simulink model "PID_Simulation_System_A"  (R2018b)
settings: Solver=VariableStepAuto  StartTime=0.0  StopTime=10  RelTol=1e-3
undefined symbols (not defined in the file): B, b, g, h, Jeq, k_noise, Kb, kd, ki, Km, kp, l, La, M, m, N, r, Ra
libraries: simulink x5, simulink_extras x1
settings Model: Creator=fred  LastModifiedBy=fredericovaz
settings SolverCC: AlgebraicLoopSolver=LineSearch
settings HardwareCC: ProdBitPerLong=64  ProdHWDeviceType=Intel->x86-64 (Linux 64)

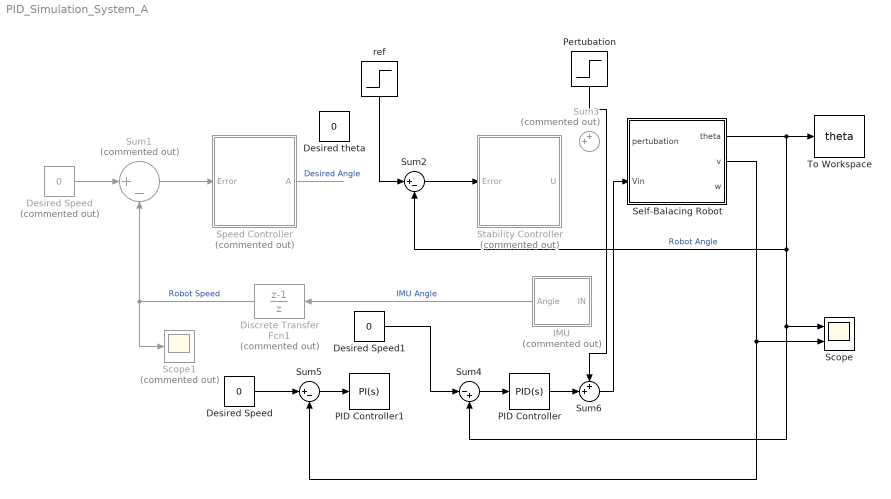
== system PID_Simulation_System_A ==
  Desired Speed : Constant  Value=0
  "Desired Speed " : Constant  Commented=on  Value=0
  Desired Speed1 : Constant  Value=0
  "Desired theta " : Constant  Value=0
  Discrete Transfer Fcn1 : DiscreteTransferFcn  Commented=on  Numerator=[1 -1]  Denominator=[1 0]  SampleTime=h
  IMU : Subsystem  Commented=on
  PID Controller : simulink/Continuous/PID Controller  Controller=PID  Form=Parallel  TimeDomain=Continuous-time  SampleTime=-1  IntegratorMethod=Forward Euler  FilterMethod=Forward Euler  ControllerParametersSource=internal  P=3218.54164072839  I=409.836899495035  D=13019.6852840674  UseFilter=on  N=3228.39836467521  TunerSelectOption=Transfer Function Based (PID Tuner App)  InitialConditionSource=internal  InitialConditionForIntegrator=0  InitialConditionForFilter=0  DifferentiatorICPrevScaledInput=0  ExternalReset=none  TrackingMode=off  Kt=1  LimitOutput=off  UpperSaturationLimit=inf  LowerSaturationLimit=-inf  LinearizeAsGain=on  AntiWindupMode=none  Kb=1  POutMin=[]  POutMax=[]  IOutMin=[]  IOutMax=[]  DOutMin=[]  DOutMax=[]  NOutMin=[]  NOutMax=[]  SumOutMin=[]  SumOutMax=[]  SaturationOutMin=[]  SaturationOutMax=[]  PParamMin=[]  PParamMax=[]  IParamMin=[]  IParamMax=[]  DParamMin=[]  DParamMax=[]  NParamMin=[]  NParamMax=[]  KbParamMin=[]  KbParamMax=[]  KtParamMin=[]  KtParamMax=[]  KbOutMin=[]  KbOutMax=[]  KtOutMin=[]  KtOutMax=[]  IntegratorOutMin=[]  IntegratorOutMax=[]  FilterOutMin=[]  FilterOutMax=[]  SumI1OutMin=[]  SumI1OutMax=[]  SumI2OutMin=[]  SumI2OutMax=[]  SumI3OutMin=[]  SumI3OutMax=[]  SumI4OutMin=[]  SumI4OutMax=[]  SumDOutMin=[]  SumDOutMax=[]  DifferentiatorOutMin=[]  DifferentiatorOutMax=[]  FilterDiffOutCoefMin=[]  FilterDiffOutCoefMax=[]  ReciprocalOutMin=[]  ReciprocalOutMax=[]  SumDenOutMin=[]  SumDenOutMax=[]  SumNumOutMin=[]  SumNumOutMax=[]  DivideOutMin=[]  DivideOutMax=[]  IntegratorContinuousStateAttributes=''  IntegratorStateMustResolveToSignalObject=off  IntegratorRTWStateStorageClass=Auto  FilterContinuousStateAttributes=''  FilterStateMustResolveToSignalObject=off  FilterRTWStateStorageClass=Auto  ParallelPVariant=InternalParameters  IdealPVariant=Disabled  IVariant=InternalParameters  DVariant=InternalParameters  IntegratorVariant=Continuous  SatVariant=Disabled  AWVariant=Passthrough  PCopyVariant=Disabled  TRVariant=Disabled  FdbkBlocksVariant=Forward  IdealPFdbkVariant=Disabled  SatFdbkVariant=Disabled  DerivativeFilterVariant=ContFilter  NVariant=InternalParameters  NCopyVariant=Disabled  FilterICVariant=InternalICsFilter  IntegratorICVariant=InternalICs  ExternalResetVariant=Disabled  TRSumVariant=Passthrough  SumFdbkVariant=Disabled  SumVariant=Sum_PID
  PID Controller1 : simulink/Continuous/PID Controller  Controller=PI  Form=Parallel  TimeDomain=Continuous-time  SampleTime=-1  IntegratorMethod=Forward Euler  FilterMethod=Forward Euler  ControllerParametersSource=internal  P=0.000483355764133952  I=1.52555105477767e-06  D=829.68075928854  UseFilter=on  N=20  TunerSelectOption=Transfer Function Based (PID Tuner App)  InitialConditionSource=internal  InitialConditionForIntegrator=0  InitialConditionForFilter=0  DifferentiatorICPrevScaledInput=0  ExternalReset=none  TrackingMode=off  Kt=1  LimitOutput=off  UpperSaturationLimit=inf  LowerSaturationLimit=-inf  LinearizeAsGain=on  AntiWindupMode=none  Kb=1  POutMin=[]  POutMax=[]  IOutMin=[]  IOutMax=[]  DOutMin=[]  DOutMax=[]  NOutMin=[]  NOutMax=[]  SumOutMin=[]  SumOutMax=[]  SaturationOutMin=[]  SaturationOutMax=[]  PParamMin=[]  PParamMax=[]  IParamMin=[]  IParamMax=[]  DParamMin=[]  DParamMax=[]  NParamMin=[]  NParamMax=[]  KbParamMin=[]  KbParamMax=[]  KtParamMin=[]  KtParamMax=[]  KbOutMin=[]  KbOutMax=[]  KtOutMin=[]  KtOutMax=[]  IntegratorOutMin=[]  IntegratorOutMax=[]  FilterOutMin=[]  FilterOutMax=[]  SumI1OutMin=[]  SumI1OutMax=[]  SumI2OutMin=[]  SumI2OutMax=[]  SumI3OutMin=[]  SumI3OutMax=[]  SumI4OutMin=[]  SumI4OutMax=[]  SumDOutMin=[]  SumDOutMax=[]  DifferentiatorOutMin=[]  DifferentiatorOutMax=[]  FilterDiffOutCoefMin=[]  FilterDiffOutCoefMax=[]  ReciprocalOutMin=[]  ReciprocalOutMax=[]  SumDenOutMin=[]  SumDenOutMax=[]  SumNumOutMin=[]  SumNumOutMax=[]  DivideOutMin=[]  DivideOutMax=[]  IntegratorContinuousStateAttributes=''  IntegratorStateMustResolveToSignalObject=off  IntegratorRTWStateStorageClass=Auto  FilterContinuousStateAttributes=''  FilterStateMustResolveToSignalObject=off  FilterRTWStateStorageClass=Auto  ParallelPVariant=InternalParameters  IdealPVariant=Disabled  IVariant=InternalParameters  DVariant=Disabled  IntegratorVariant=Continuous  SatVariant=Disabled  AWVariant=Passthrough  PCopyVariant=Disabled  TRVariant=Disabled  FdbkBlocksVariant=Forward  IdealPFdbkVariant=Disabled  SatFdbkVariant=Disabled  DerivativeFilterVariant=Disabled  NVariant=Disabled  NCopyVariant=Disabled_SignalSpec  FilterICVariant=Disabled  IntegratorICVariant=InternalICs  ExternalResetVariant=Disabled  TRSumVariant=Passthrough  SumFdbkVariant=Disabled  SumVariant=Sum_PI
  Pertubation : Step  Time=2  After=15
  Scope : Scope  NumInputPorts=2
  Scope1 : Scope  Commented=on
  Self-Balacing Robot : Subsystem
  Speed Controller : Subsystem  Commented=on
  Stability Controller : Subsystem  Commented=on
  Sum1 : Sum  Commented=on  Inputs=|+-
  Sum2 : Sum  Inputs=|+-
  Sum3 : Sum  Commented=on  Inputs=++|
  Sum4 : Sum  Inputs=|-+
  Sum5 : Sum  Inputs=|+-
  Sum6 : Sum  Inputs=++|
  To Workspace : ToWorkspace  VariableName=theta  SaveFormat=Timeseries  SampleTime=-1
      settings: Save2DSignal=2-D array (concatenate along first dimension)
  ref : Step  Time=2  After=0.25  SampleTime=h
  wires:
  IMU/1(Angle) -> Discrete Transfer Fcn1/1  "IMU Angle"
  Self-Balacing Robot/1(theta) -> To Workspace/1, Sum2/2, Scope/1, Sum4/2  "Robot Angle"
  Speed Controller/1(A) -> ?  "Desired Angle"
  Sum1/1 -> Speed Controller/1(Error)
  "Desired Speed "/1 -> Sum1/1
  Discrete Transfer Fcn1/1 -> Scope1/1, Sum1/2  "Robot Speed"
  Sum2/1 -> Stability Controller/1(Error)
  ref/1 -> Sum2/1
  Sum4/1 -> PID Controller/1
  Sum5/1 -> PID Controller1/1
  Self-Balacing Robot/2(v) -> Scope/2, Sum5/2
  PID Controller/1 -> Sum6/2
  Sum6/1 -> Self-Balacing Robot/2(Vin)
  Pertubation/1 -> Sum6/1
  Desired Speed/1 -> Sum5/1
  Desired Speed1/1 -> Sum4/1

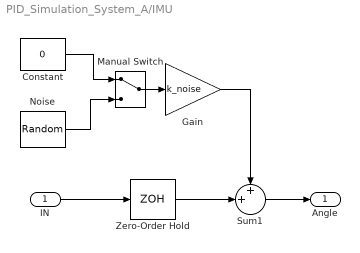
== system PID_Simulation_System_A/IMU ==
  IN : Inport
  Constant : Constant  Value=0
  Gain : Gain  Gain=k_noise
  Manual Switch : ManualSwitch
  Noise : UniformRandomNumber  Minimum=-0.1  Maximum=0.1  SampleTime=h
  Sum1 : Sum  Inputs=++|
  Zero-Order Hold : ZeroOrderHold  SampleTime=h
  Angle : Outport
  wires:
  IN/1 -> Zero-Order Hold/1
  Constant/1 -> Manual Switch/1
  Noise/1 -> Manual Switch/2
  Manual Switch/1 -> Gain/1
  Gain/1 -> Sum1/1
  Zero-Order Hold/1 -> Sum1/2
  Sum1/1 -> Angle/1

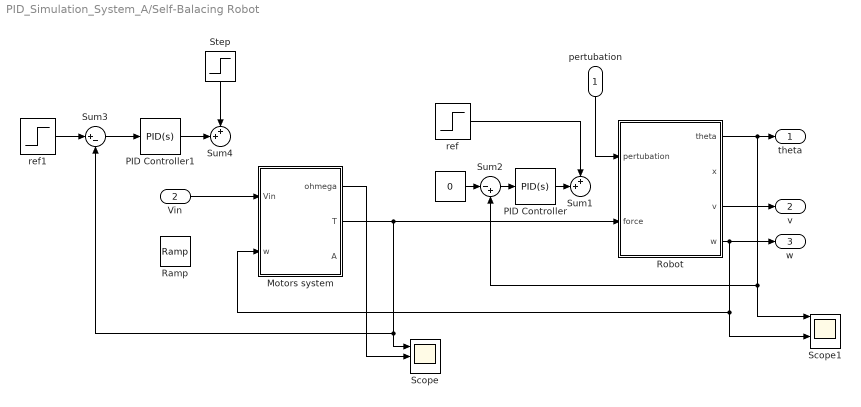
== system PID_Simulation_System_A/Self-Balacing Robot ==
  pertubation : Inport
  Vin : Inport  Port=2
  " " : Constant  Value=0
  Motors system : Subsystem
  PID Controller : simulink/Continuous/PID Controller  Controller=PID  Form=Parallel  TimeDomain=Continuous-time  SampleTime=-1  IntegratorMethod=Forward Euler  FilterMethod=Forward Euler  ControllerParametersSource=internal  P=6572.38369505498  I=1124.56192224529  D=829.68075928854  UseFilter=on  N=20  TunerSelectOption=Transfer Function Based (PID Tuner App)  InitialConditionSource=internal  InitialConditionForIntegrator=0  InitialConditionForFilter=0  DifferentiatorICPrevScaledInput=0  ExternalReset=none  TrackingMode=off  Kt=1  LimitOutput=off  UpperSaturationLimit=inf  LowerSaturationLimit=-inf  LinearizeAsGain=on  AntiWindupMode=none  Kb=1  POutMin=[]  POutMax=[]  IOutMin=[]  IOutMax=[]  DOutMin=[]  DOutMax=[]  NOutMin=[]  NOutMax=[]  SumOutMin=[]  SumOutMax=[]  SaturationOutMin=[]  SaturationOutMax=[]  PParamMin=[]  PParamMax=[]  IParamMin=[]  IParamMax=[]  DParamMin=[]  DParamMax=[]  NParamMin=[]  NParamMax=[]  KbParamMin=[]  KbParamMax=[]  KtParamMin=[]  KtParamMax=[]  KbOutMin=[]  KbOutMax=[]  KtOutMin=[]  KtOutMax=[]  IntegratorOutMin=[]  IntegratorOutMax=[]  FilterOutMin=[]  FilterOutMax=[]  SumI1OutMin=[]  SumI1OutMax=[]  SumI2OutMin=[]  SumI2OutMax=[]  SumI3OutMin=[]  SumI3OutMax=[]  SumI4OutMin=[]  SumI4OutMax=[]  SumDOutMin=[]  SumDOutMax=[]  DifferentiatorOutMin=[]  DifferentiatorOutMax=[]  FilterDiffOutCoefMin=[]  FilterDiffOutCoefMax=[]  ReciprocalOutMin=[]  ReciprocalOutMax=[]  SumDenOutMin=[]  SumDenOutMax=[]  SumNumOutMin=[]  SumNumOutMax=[]  DivideOutMin=[]  DivideOutMax=[]  IntegratorContinuousStateAttributes=''  IntegratorStateMustResolveToSignalObject=off  IntegratorRTWStateStorageClass=Auto  FilterContinuousStateAttributes=''  FilterStateMustResolveToSignalObject=off  FilterRTWStateStorageClass=Auto  ParallelPVariant=InternalParameters  IdealPVariant=Disabled  IVariant=InternalParameters  DVariant=InternalParameters  IntegratorVariant=Continuous  SatVariant=Disabled  AWVariant=Passthrough  PCopyVariant=Disabled  TRVariant=Disabled  FdbkBlocksVariant=Forward  IdealPFdbkVariant=Disabled  SatFdbkVariant=Disabled  DerivativeFilterVariant=ContFilter  NVariant=InternalParameters  NCopyVariant=Disabled  FilterICVariant=InternalICsFilter  IntegratorICVariant=InternalICs  ExternalResetVariant=Disabled  TRSumVariant=Passthrough  SumFdbkVariant=Disabled  SumVariant=Sum_PID
  PID Controller1 : simulink/Continuous/PID Controller  Controller=PID  Form=Parallel  TimeDomain=Continuous-time  SampleTime=-1  IntegratorMethod=Forward Euler  FilterMethod=Forward Euler  ControllerParametersSource=internal  P=6.37249058786852  I=20.4430705513798  D=0.210868925442999  UseFilter=on  N=10.486281731924  TunerSelectOption=Transfer Function Based (PID Tuner App)  InitialConditionSource=internal  InitialConditionForIntegrator=0  InitialConditionForFilter=0  DifferentiatorICPrevScaledInput=0  ExternalReset=none  TrackingMode=off  Kt=1  LimitOutput=off  UpperSaturationLimit=inf  LowerSaturationLimit=-inf  LinearizeAsGain=on  AntiWindupMode=none  Kb=1  POutMin=[]  POutMax=[]  IOutMin=[]  IOutMax=[]  DOutMin=[]  DOutMax=[]  NOutMin=[]  NOutMax=[]  SumOutMin=[]  SumOutMax=[]  SaturationOutMin=[]  SaturationOutMax=[]  PParamMin=[]  PParamMax=[]  IParamMin=[]  IParamMax=[]  DParamMin=[]  DParamMax=[]  NParamMin=[]  NParamMax=[]  KbParamMin=[]  KbParamMax=[]  KtParamMin=[]  KtParamMax=[]  KbOutMin=[]  KbOutMax=[]  KtOutMin=[]  KtOutMax=[]  IntegratorOutMin=[]  IntegratorOutMax=[]  FilterOutMin=[]  FilterOutMax=[]  SumI1OutMin=[]  SumI1OutMax=[]  SumI2OutMin=[]  SumI2OutMax=[]  SumI3OutMin=[]  SumI3OutMax=[]  SumI4OutMin=[]  SumI4OutMax=[]  SumDOutMin=[]  SumDOutMax=[]  DifferentiatorOutMin=[]  DifferentiatorOutMax=[]  FilterDiffOutCoefMin=[]  FilterDiffOutCoefMax=[]  ReciprocalOutMin=[]  ReciprocalOutMax=[]  SumDenOutMin=[]  SumDenOutMax=[]  SumNumOutMin=[]  SumNumOutMax=[]  DivideOutMin=[]  DivideOutMax=[]  IntegratorContinuousStateAttributes=''  IntegratorStateMustResolveToSignalObject=off  IntegratorRTWStateStorageClass=Auto  FilterContinuousStateAttributes=''  FilterStateMustResolveToSignalObject=off  FilterRTWStateStorageClass=Auto  ParallelPVariant=InternalParameters  IdealPVariant=Disabled  IVariant=InternalParameters  DVariant=InternalParameters  IntegratorVariant=Continuous  SatVariant=Disabled  AWVariant=Passthrough  PCopyVariant=Disabled  TRVariant=Disabled  FdbkBlocksVariant=Forward  IdealPFdbkVariant=Disabled  SatFdbkVariant=Disabled  DerivativeFilterVariant=ContFilter  NVariant=InternalParameters  NCopyVariant=Disabled  FilterICVariant=InternalICsFilter  IntegratorICVariant=InternalICs  ExternalResetVariant=Disabled  TRSumVariant=Passthrough  SumFdbkVariant=Disabled  SumVariant=Sum_PID
  Ramp : simulink/Sources/Ramp  slope=1  start=2  InitialOutput=0
  Robot : Subsystem
  Scope : Scope  NumInputPorts=3
  Scope1 : Scope  NumInputPorts=4
  Step : Step  After=12  SampleTime=0
  Sum1 : Sum  Inputs=++|
  Sum2 : Sum  Inputs=|-+
  Sum3 : Sum  Inputs=|+-
  Sum4 : Sum  Inputs=++|
  ref : Step  Time=2  After=15
  ref1 : Step  Time=2  After=0.25  SampleTime=h
  theta : Outport
  v : Outport  Port=2
  w : Outport  Port=3
  wires:
  Robot/1(theta) -> Scope1/1, Sum2/2, theta/1
  Robot/3(v) -> v/1
  Robot/4(w) -> w/1, Scope1/3, Motors system/2(w)
  Motors system/2(T) -> Sum3/2, Scope/1, Robot/2(force)
  Motors system/1(ohmega) -> Scope/2
  Sum2/1 -> PID Controller/1
  " "/1 -> Sum2/1
  PID Controller/1 -> Sum1/2
  ref/1 -> Sum1/1
  PID Controller1/1 -> Sum4/2
  pertubation/1 -> Robot/1(pertubation)
  Sum3/1 -> PID Controller1/1
  ref1/1 -> Sum3/1
  Step/1 -> Sum4/1
  Vin/1 -> Motors system/1(Vin)

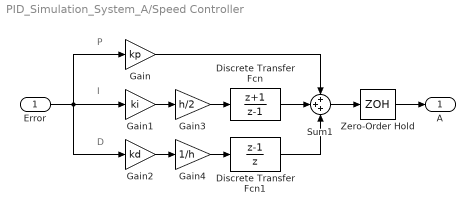
== system PID_Simulation_System_A/Speed Controller ==
  note: I
  note: D
  note: P
  Error : Inport
  Discrete Transfer Fcn : DiscreteTransferFcn  Numerator=[1 +1]  Denominator=[1 -1]  SampleTime=h
  Discrete Transfer Fcn1 : DiscreteTransferFcn  Numerator=[1 -1]  Denominator=[1 0]  SampleTime=h
  Gain : Gain  Gain=kp
  Gain1 : Gain  Gain=ki
  Gain2 : Gain  Gain=kd
  Gain3 : Gain  Gain=h/2
  Gain4 : Gain  Gain=1/h
  Sum1 : Sum  Inputs=+++
  Zero-Order Hold : ZeroOrderHold  SampleTime=h
  A : Outport
  wires:
  Gain1/1 -> Gain3/1
  Error/1 -> Gain1/1, Gain2/1, Gain/1
  Zero-Order Hold/1 -> A/1
  Sum1/1 -> Zero-Order Hold/1
  Gain2/1 -> Gain4/1
  Gain/1 -> Sum1/1
  Gain3/1 -> Discrete Transfer Fcn/1
  Discrete Transfer Fcn/1 -> Sum1/2
  Gain4/1 -> Discrete Transfer Fcn1/1
  Discrete Transfer Fcn1/1 -> Sum1/3

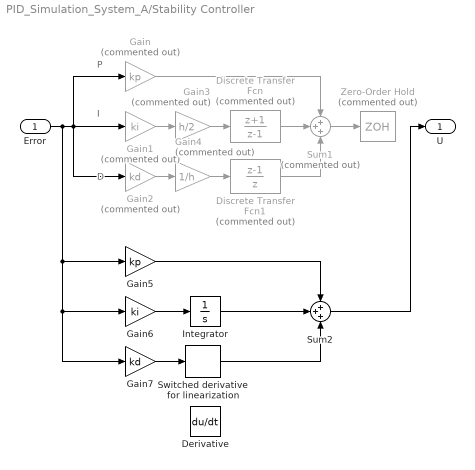
== system PID_Simulation_System_A/Stability Controller ==
  note: I
  note: D
  note: P
  Error : Inport
  Derivative : Derivative
  Discrete Transfer Fcn : DiscreteTransferFcn  Commented=on  Numerator=[1 +1]  Denominator=[1 -1]  SampleTime=h
  Discrete Transfer Fcn1 : DiscreteTransferFcn  Commented=on  Numerator=[1 -1]  Denominator=[1 0]  SampleTime=h
  Gain : Gain  Commented=on  Gain=kp
  Gain1 : Gain  Commented=on  Gain=ki
  Gain2 : Gain  Commented=on  Gain=kd
  Gain3 : Gain  Commented=on  Gain=h/2
  Gain4 : Gain  Commented=on  Gain=1/h
  Gain5 : Gain  Gain=kp
  Gain6 : Gain  Gain=ki
  Gain7 : Gain  Gain=kd
  Integrator : Integrator
  Sum1 : Sum  Commented=on  Inputs=+++
  Sum2 : Sum  Inputs=+++
  Switched derivative for linearization : simulink_extras/Linearization/Switched derivative for linearization  switchVal=0  derivConst=100
      settings: SourceProductName=Simulink  SourceProductBaseCode=SL
  Zero-Order Hold : ZeroOrderHold  Commented=on  SampleTime=h
  U : Outport
  wires:
  Gain1/1 -> Gain3/1
  Error/1 -> Gain5/1, Gain6/1, Gain7/1, Gain1/1, Gain2/1, Gain/1
  Sum1/1 -> Zero-Order Hold/1
  Gain2/1 -> Gain4/1
  Gain/1 -> Sum1/1
  Gain3/1 -> Discrete Transfer Fcn/1
  Discrete Transfer Fcn/1 -> Sum1/2
  Gain4/1 -> Discrete Transfer Fcn1/1
  Discrete Transfer Fcn1/1 -> Sum1/3
  Sum2/1 -> U/1
  Gain7/1 -> Switched derivative for linearization/1
  Gain6/1 -> Integrator/1
  Integrator/1 -> Sum2/2
  Switched derivative for linearization/1 -> Sum2/3
  Gain5/1 -> Sum2/1

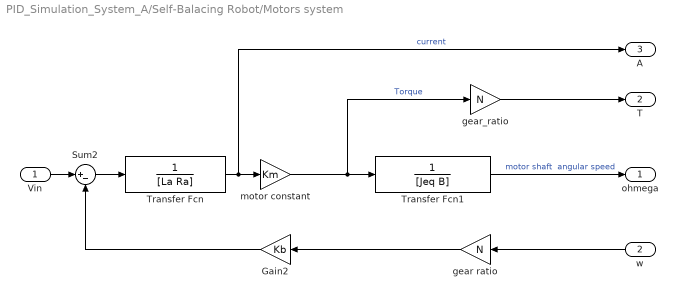
== system PID_Simulation_System_A/Self-Balacing Robot/Motors system ==
  Vin : Inport
  w : Inport  Port=2
  Gain2 : Gain  Gain=Kb
  Sum2 : Sum  Inputs=|+-
  Transfer Fcn : TransferFcn  Denominator=[La Ra]
  Transfer Fcn1 : TransferFcn  Denominator=[Jeq B]
  gear ratio : Gain  Gain=N
  gear_ratio : Gain  Gain=N
  motor constant : Gain  Gain=Km
  ohmega : Outport
  T : Outport  Port=2
  A : Outport  Port=3
  wires:
  gear ratio/1 -> Gain2/1
  motor constant/1 -> gear_ratio/1, Transfer Fcn1/1  "Torque"
  Transfer Fcn/1 -> A/1, motor constant/1  "current"
  gear_ratio/1 -> T/1
  Gain2/1 -> Sum2/2
  w/1 -> gear ratio/1
  Vin/1 -> Sum2/1
  Sum2/1 -> Transfer Fcn/1
  Transfer Fcn1/1 -> ohmega/1  "motor shaft  angular speed"

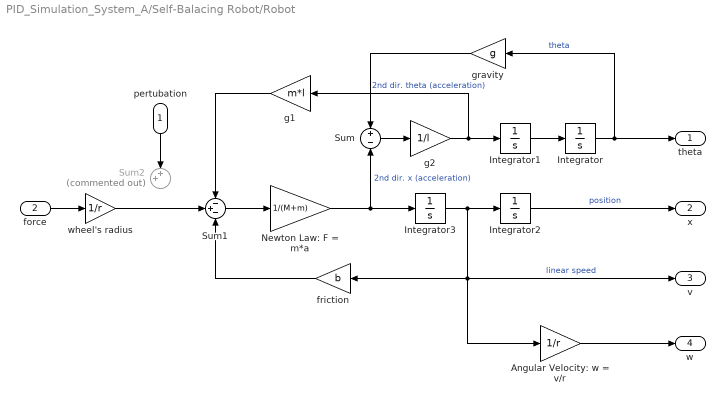
== system PID_Simulation_System_A/Self-Balacing Robot/Robot ==
  pertubation : Inport
  force : Inport  Port=2
  Angular Velocity: w = v/r : Gain  Gain=1/r
  Integrator{,1..3} (4 alike) : Integrator
  Newton Law: F = m*a : Gain  Gain=1/(M+m)
  Sum : Sum  Inputs=+-
  Sum1 : Sum  Inputs=-+-
  Sum2 : Sum  Commented=on  Inputs=++|
  friction : Gain  Gain=b
  g1 : Gain  Gain=m*l
  g2 : Gain  Gain=1/l
  gravity : Gain  Gain=g
  wheel's radius : Gain  Gain=1/r
  theta : Outport
  x : Outport  Port=2
  v : Outport  Port=3
  w : Outport  Port=4
  wires:
  Sum/1 -> g2/1
  Integrator1/1 -> Integrator/1
  Integrator2/1 -> x/1  "position"
  Sum1/1 -> Newton Law: F = m*a/1
  Newton Law: F = m*a/1 -> Sum/2, Integrator3/1  "2nd dir. x (acceleration)"
  friction/1 -> Sum1/3
  pertubation/1 -> Sum2/1
  Integrator3/1 -> v/1, Angular Velocity: w = v/r/1, friction/1, Integrator2/1  "linear speed"
  g2/1 -> g1/1, Integrator1/1  "2nd dir. theta (acceleration)"
  g1/1 -> Sum1/1
  Integrator/1 -> gravity/1, theta/1  "theta"
  Angular Velocity: w = v/r/1 -> w/1
  force/1 -> wheel's radius/1
  wheel's radius/1 -> Sum1/2
  gravity/1 -> Sum/1
